simulink model "MotorParameterIdentification_SIM"  (R2017b)
settings: Solver=FixedStepAuto  StartTime=0.0  StopTime=100  FixedStep=0.001  RelTol=1e-3
values from neighbouring files (symbols this model uses):
  Cpsi = 3.77890170629e-05    [MotorParameter.mat]    (also in ParameterInit.m = 3e-05)
  IR = 0.00135926825474    [MotorParameter.mat]    (also in ParameterInit.m = 0.00012)
  uR_0 = ur(1)    [ParameterInit.m]
undefined symbols (not defined in the file or in its folder): magnitude
settings Model: Creator=michael  LastModifiedBy=michael

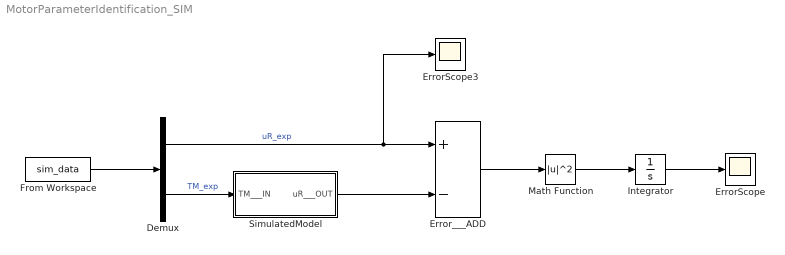
== system MotorParameterIdentification_SIM ==
  Demux : Demux  Outputs=2
  ErrorScope : Scope
  ErrorScope3 : Scope
  Error___ADD : Sum  Inputs=+-
  From Workspace : FromWorkspace  VariableName=sim_data  SampleTime=0.01
  Integrator : Integrator
  Math Function : Math  Operator=magnitude^2  SaturateOnIntegerOverflow=on
  SimulatedModel : Subsystem
  wires:
  From Workspace/1 -> Demux/1
  Demux/2 -> SimulatedModel/1(TM___IN)  "TM_exp"
  SimulatedModel/1(uR___OUT) -> Error___ADD/2
  Demux/1 -> ErrorScope3/1, Error___ADD/1  "uR_exp"
  Error___ADD/1 -> Math Function/1
  Math Function/1 -> Integrator/1
  Integrator/1 -> ErrorScope/1

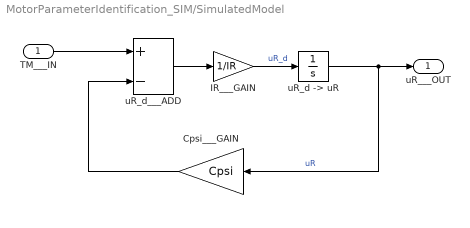
== system MotorParameterIdentification_SIM/SimulatedModel ==
  TM___IN : Inport
  Cpsi___GAIN : Gain  Gain=Cpsi
  IR___GAIN : Gain  Gain=1/IR
  "uR_d -> uR" : Integrator  InitialCondition=uR_0
  uR_d___ADD : Sum  Inputs=+-
  uR___OUT : Outport
  wires:
  "uR_d -> uR"/1 -> Cpsi___GAIN/1, uR___OUT/1  "uR"
  TM___IN/1 -> uR_d___ADD/1
  uR_d___ADD/1 -> IR___GAIN/1
  IR___GAIN/1 -> "uR_d -> uR"/1  "uR_d"
  Cpsi___GAIN/1 -> uR_d___ADD/2
